simulink model "FirmwareController"  (R2022a)
settings: Solver=FixedStepDiscrete  StartTime=0.0  StopTime=10.0  RelTol=1e-3
model workspace (MAT data in the model file):
  HighLevel = Simulink.Bus
  HighLevel.Alignment = -1
  HighLevel.PreserveElementDimensions = 0
  HighLevel.Elements_internal(1) = Simulink.BusElement
  HighLevel.Elements_internal(1).DimensionsMode = 'Fixed'
  HighLevel.Elements_internal(1).SamplingMode = 'Sample based'
  HighLevel.Elements_internal(1).SampleTime = -1
  HighLevel.Elements_internal(1).Name = 'VelocityCommand'
  HighLevel.Elements_internal(1).DataType_internal = 'double'
  HighLevel.Elements_internal(1).Complexity = 'real'
  HighLevel.Elements_internal(1).Dimensions = 1
  HighLevel.Elements_internal(2) = Simulink.BusElement
  HighLevel.Elements_internal(2).DimensionsMode = 'Fixed'
  HighLevel.Elements_internal(2).SamplingMode = 'Sample based'
  HighLevel.Elements_internal(2).SampleTime = -1
  HighLevel.Elements_internal(2).Name = 'Odometry'
  HighLevel.Elements_internal(2).DataType_internal = 'double'
  HighLevel.Elements_internal(2).Complexity = 'real'
  HighLevel.Elements_internal(2).Dimensions = 1
  HighLevel.Elements_internal(3) = Simulink.BusElement
  HighLevel.Elements_internal(3).DimensionsMode = 'Fixed'
  HighLevel.Elements_internal(3).SamplingMode = 'Sample based'
  HighLevel.Elements_internal(3).SampleTime = -1
  HighLevel.Elements_internal(3).Name = 'ManipulatorTrajectory'
  HighLevel.Elements_internal(3).DataType_internal = 'double'
  HighLevel.Elements_internal(3).Complexity = 'real'
  HighLevel.Elements_internal(3).Dimensions = 1
  HighLevel.DataScope = 'Auto'
  ManipulatorSensorData = Simulink.Bus
  ManipulatorSensorData.Alignment = -1
  ManipulatorSensorData.PreserveElementDimensions = 0
  ManipulatorSensorData.Elements_internal(1) = Simulink.BusElement
  ManipulatorSensorData.Elements_internal(1).DimensionsMode = 'Fixed'
  ManipulatorSensorData.Elements_internal(1).SamplingMode = 'Sample based'
  ManipulatorSensorData.Elements_internal(1).SampleTime = -1
  ManipulatorSensorData.Elements_internal(1).Name = 'EncoderJoint1'
  ManipulatorSensorData.Elements_internal(1).DataType_internal = 'double'
  ManipulatorSensorData.Elements_internal(1).Complexity = 'real'
  ManipulatorSensorData.Elements_internal(1).Dimensions = 1
  ManipulatorSensorData.Elements_internal(2) = Simulink.BusElement
  ManipulatorSensorData.Elements_internal(2).DimensionsMode = 'Fixed'
  ManipulatorSensorData.Elements_internal(2).SamplingMode = 'Sample based'
  ManipulatorSensorData.Elements_internal(2).SampleTime = -1
  ManipulatorSensorData.Elements_internal(2).Name = 'EncoderJoint2'
  ManipulatorSensorData.Elements_internal(2).DataType_internal = 'double'
  ManipulatorSensorData.Elements_internal(2).Complexity = 'real'
  ManipulatorSensorData.Elements_internal(2).Dimensions = 1
  ManipulatorSensorData.Elements_internal(3) = Simulink.BusElement
  ManipulatorSensorData.Elements_internal(3).DimensionsMode = 'Fixed'
  ManipulatorSensorData.Elements_internal(3).SamplingMode = 'Sample based'
  ManipulatorSensorData.Elements_internal(3).SampleTime = -1
  ManipulatorSensorData.Elements_internal(3).Name = 'EncoderJoint3'
  ManipulatorSensorData.Elements_internal(3).DataType_internal = 'double'
  ManipulatorSensorData.Elements_internal(3).Complexity = 'real'
  ManipulatorSensorData.Elements_internal(3).Dimensions = 1
  ManipulatorSensorData.Elements_internal(4) = Simulink.BusElement
  ManipulatorSensorData.Elements_internal(4).DimensionsMode = 'Fixed'
  ManipulatorSensorData.Elements_internal(4).SamplingMode = 'Sample based'
  ManipulatorSensorData.Elements_internal(4).SampleTime = -1
  ManipulatorSensorData.Elements_internal(4).Name = 'EncoderJoint4'
  ManipulatorSensorData.Elements_internal(4).DataType_internal = 'double'
  ManipulatorSensorData.Elements_internal(4).Complexity = 'real'
  ManipulatorSensorData.Elements_internal(4).Dimensions = 1
  ManipulatorSensorData.Elements_internal(5) = Simulink.BusElement
  ManipulatorSensorData.Elements_internal(5).DimensionsMode = 'Fixed'
  ManipulatorSensorData.Elements_internal(5).SamplingMode = 'Sample based'
  ManipulatorSensorData.Elements_internal(5).SampleTime = -1
  ManipulatorSensorData.Elements_internal(5).Name = 'EncoderJoint5'
  ManipulatorSensorData.Elements_internal(5).DataType_internal = 'double'
  ManipulatorSensorData.Elements_internal(5).Complexity = 'real'
  ManipulatorSensorData.Elements_internal(5).Dimensions = 1
  ManipulatorSensorData.Elements_internal(6) = Simulink.BusElement
  ManipulatorSensorData.Elements_internal(6).DimensionsMode = 'Fixed'
  ManipulatorSensorData.Elements_internal(6).SamplingMode = 'Sample based'
  ManipulatorSensorData.Elements_internal(6).SampleTime = -1
  ManipulatorSensorData.Elements_internal(6).Name = 'EncoderJoint6'
  ManipulatorSensorData.Elements_internal(6).DataType_internal = 'double'
  ManipulatorSensorData.Elements_internal(6).Complexity = 'real'
  ManipulatorSensorData.Elements_internal(6).Dimensions = 1
  ManipulatorSensorData.Elements_internal(7) = Simulink.BusElement
  ManipulatorSensorData.Elements_internal(7).DimensionsMode = 'Fixed'
  ManipulatorSensorData.Elements_internal(7).SamplingMode = 'Sample based'
  ManipulatorSensorData.Elements_internal(7).SampleTime = -1
  ManipulatorSensorData.Elements_internal(7).Name = 'EncoderJoint7'
  ManipulatorSensorData.Elements_internal(7).DataType_internal = 'double'
  ManipulatorSensorData.Elements_internal(7).Complexity = 'real'
  ManipulatorSensorData.Elements_internal(7).Dimensions = 1
  ManipulatorSensorData.DataScope = 'Auto'
  MobileBaseSensorData = Simulink.Bus
  MobileBaseSensorData.Alignment = -1
  MobileBaseSensorData.PreserveElementDimensions = 0
  MobileBaseSensorData.Elements_internal(1) = Simulink.BusElement
  MobileBaseSensorData.Elements_internal(1).DimensionsMode = 'Fixed'
  MobileBaseSensorData.Elements_internal(1).SamplingMode = 'Sample based'
  MobileBaseSensorData.Elements_internal(1).SampleTime = -1
  MobileBaseSensorData.Elements_internal(1).Name = 'EncoderMotorL'
  MobileBaseSensorData.Elements_internal(1).DataType_internal = 'double'
  MobileBaseSensorData.Elements_internal(1).Complexity = 'real'
  MobileBaseSensorData.Elements_internal(1).Dimensions = 1
  MobileBaseSensorData.Elements_internal(2) = Simulink.BusElement
  MobileBaseSensorData.Elements_internal(2).DimensionsMode = 'Fixed'
  MobileBaseSensorData.Elements_internal(2).SamplingMode = 'Sample based'
  MobileBaseSensorData.Elements_internal(2).SampleTime = -1
  MobileBaseSensorData.Elements_internal(2).Name = 'EncoderMotorR'
  MobileBaseSensorData.Elements_internal(2).DataType_internal = 'double'
  MobileBaseSensorData.Elements_internal(2).Complexity = 'real'
  MobileBaseSensorData.Elements_internal(2).Dimensions = 1
  MobileBaseSensorData.Elements_internal(3) = Simulink.BusElement
  MobileBaseSensorData.Elements_internal(3).DimensionsMode = 'Fixed'
  MobileBaseSensorData.Elements_internal(3).SamplingMode = 'Sample based'
  MobileBaseSensorData.Elements_internal(3).SampleTime = -1
  MobileBaseSensorData.Elements_internal(3).Name = 'IMU'
  MobileBaseSensorData.Elements_internal(3).DataType_internal = 'double'
  MobileBaseSensorData.Elements_internal(3).Complexity = 'real'
  MobileBaseSensorData.Elements_internal(3).Dimensions = 1
  MobileBaseSensorData.DataScope = 'Auto'
settings Model: Creator=EarthPhisek  LastModifiedBy=EarthPhisek
settings OptimizationCC: EnhancedBackFolding=on  PassReuseOutputArgsAs=Individual arguments  ZeroExternalMemoryAtStartup=off  ZeroInternalMemoryAtStartup=off  MaxStackSize=64  OptimizeBlockOrder=speed  DifferentSizesBufferReuse=on  OptimizationCustomize=off  EfficientTunableParamExpr=on
settings DebuggingCC: ParameterTunabilityLossMsg=error
settings HardwareCC: UseEmbeddedCoderFeatures=off
settings SFSimCC: MATLABDynamicMemAlloc=off
settings RTWCC: SystemTargetFile=ert.tlc  HardwareBoard=Robot Operating System 2 (ROS 2)  TLCOptions="-aInlineSetEventsForThisBaseRateFcn=TLC_FALSE -aSuppressMultiTaskScheduler=TLC_FALSE  -aRateBasedStepFcn=0"  TemplateMakefile=ert_default_tmf  Toolchain=Colcon Tools  TargetLang=C++
settings CodeAppCC: ForceParamTrailComments=on  IgnoreCustomStorageClasses=off  OperatorAnnotations=on  SimulinkDataObjDesc=on  SFDataObjDesc=on  InsertBlockDesc=on
settings ERTTargetCC: CodeInterfacePackaging=C++ class  SupportNonInlinedSFcns=on  RootIOFormat=Structure reference

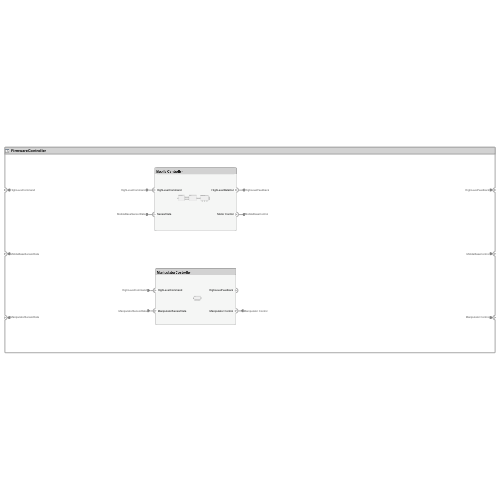
[thumbnail: Simulink's stored preview of the top-level diagram]
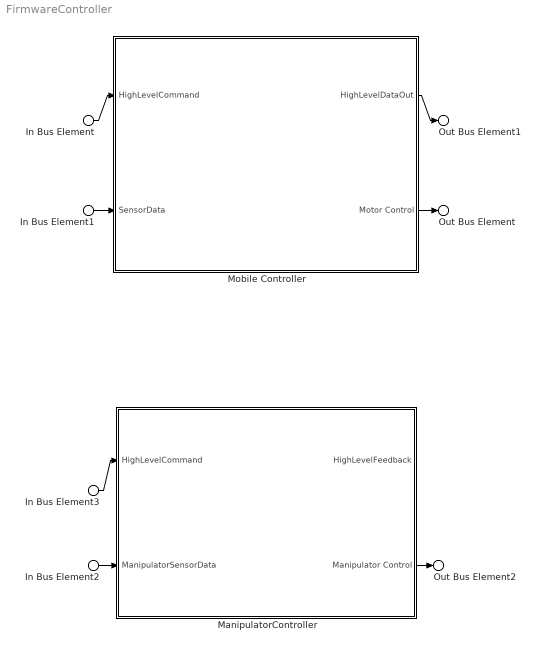
== system FirmwareController ==
  In Bus Element : Inport  PortName=HighLevelCommand
  In Bus Element3 : Inport  PortName=HighLevelCommand
  In Bus Element1 : Inport  Port=2  PortName=MobileBaseSensorData
  In Bus Element2 : Inport  Port=3  PortName=ManipulatorSensorData
  ManipulatorController : Subsystem
      settings: PortSchema="{\"entries\":[{\"content\":{\"headerSize\":26,\"margin\":15,\"minimumSpacing\":25,\"sides\":[{\"content\":{\"connectorIds\":[\"In1\",\"In2\"]},\"type\":\"ConnectorPlacement.EquallySpacedRectSide\",\"uuid\":\"c98ff4be-64d0-449e-9b1d-a8301930c005\"},{\"content\":{\"connectorIds\":[\"Out1\",\"Out2\"],\"side\":\"RIGHT\"},\"type\":\"ConnectorPlacement.EquallySpacedRectSide\",\"uuid\":\"687eed08-6ff3-4e87-827e-4ed9dc740528\"},{\"content\":{\"connectorIds\":[],\"side\":\"TOP\"},\"type\":\"ConnectorPlacement.EquallySpacedRectSide\",\"uuid\":\"c1e53efb-7b04-4802-8059-06db2c482b4f\"}]},\"type\":\"ConnectorPlacement.EquallySpacedConnector\",\"uuid\":\"21e22d49-20f6-4ec3-b79a-f2c75a9aa23d\"}],\"packageUris\":[\"http://schema.mathworks.com/mf0/Connector/R2020b\"],\"version\":\"1.0\"}"
  Mobile Controller : Subsystem
      settings: PortSchema="{\"entries\":[{\"content\":{\"headerSize\":26,\"margin\":15,\"minimumSpacing\":25,\"sides\":[{\"content\":{\"connectorIds\":[\"In1\",\"In2\"]},\"type\":\"ConnectorPlacement.EquallySpacedRectSide\",\"uuid\":\"dd41dd12-49ec-4c74-984d-ae398e001f17\"},{\"content\":{\"connectorIds\":[\"Out1\",\"Out2\"],\"side\":\"RIGHT\"},\"type\":\"ConnectorPlacement.EquallySpacedRectSide\",\"uuid\":\"7b6711d5-260d-4adb-8390-dd0a2fe64eed\"},{\"content\":{\"connectorIds\":[],\"side\":\"TOP\"},\"type\":\"ConnectorPlacement.EquallySpacedRectSide\",\"uuid\":\"51c2854e-5efe-4dec-8c07-70731026f3e8\"}]},\"type\":\"ConnectorPlacement.EquallySpacedConnector\",\"uuid\":\"aa3377b9-5458-4828-a095-24c10dd42ea0\"}],\"packageUris\":[\"http://schema.mathworks.com/mf0/Connector/R2020b\"],\"version\":\"1.0\"}"
  Out Bus Element1 : Outport  PortName=HighLevelFeedback
  Out Bus Element : Outport  Port=2  PortName=MobileBaseControl
  Out Bus Element2 : Outport  Port=3  PortName=Manipulator Control
  wires:
  In Bus Element1/1 -> Mobile Controller/2(SensorData)
  In Bus Element/1 -> Mobile Controller/1(HighLevelCommand)
  In Bus Element2/1 -> ManipulatorController/2(ManipulatorSensorData)
  In Bus Element3/1 -> ManipulatorController/1(HighLevelCommand)
  Mobile Controller/2(Motor Control) -> Out Bus Element/1
  Mobile Controller/1(HighLevelDataOut) -> Out Bus Element1/1
  ManipulatorController/2(Manipulator Control) -> Out Bus Element2/1

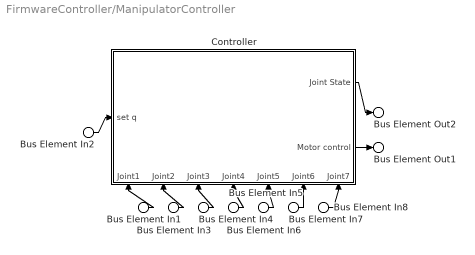
== system FirmwareController/ManipulatorController ==
  Bus Element In2 : Inport  PortName=HighLevelCommand  Element=ManipulatorTrajectory
  Bus Element In1 : Inport  Port=2  PortName=ManipulatorSensorData  Element=EncoderJoint1
  Bus Element In3 : Inport  Port=2  PortName=ManipulatorSensorData  Element=EncoderJoint2
  Bus Element In4 : Inport  Port=2  PortName=ManipulatorSensorData  Element=EncoderJoint3
  Bus Element In5 : Inport  Port=2  PortName=ManipulatorSensorData  Element=EncoderJoint4
  Bus Element In6 : Inport  Port=2  PortName=ManipulatorSensorData  Element=EncoderJoint5
  Bus Element In7 : Inport  Port=2  PortName=ManipulatorSensorData  Element=EncoderJoint6
  Bus Element In8 : Inport  Port=2  PortName=ManipulatorSensorData  Element=EncoderJoint7
  Controller : Subsystem
      settings: PortSchema="{\"entries\":[{\"content\":{\"headerSize\":26,\"margin\":15,\"minimumSpacing\":25,\"sides\":[{\"content\":{\"connectorIds\":[\"In8\"]},\"type\":\"ConnectorPlacement.EquallySpacedRectSide\",\"uuid\":\"c98ff4be-64d0-449e-9b1d-a8301930c005\"},{\"content\":{\"connectorIds\":[\"Out1\",\"Out2\"],\"side\":\"RIGHT\"},\"type\":\"ConnectorPlacement.EquallySpacedRectSide\",\"uuid\":\"687eed08-6ff3-4e87-827e-4ed9dc740528\"},{\"content\":{\"connectorIds\":[],\"side\":\"TOP\"},\"type\":\"ConnectorPlacement.EquallySpacedRectSide\",\"uuid\":\"c1e53efb-7b04-4802-8059-06db2c482b4f\"},{\"content\":{\"connectorIds\":[\"In1\",\"In2\",\"In3\",\"In4\",\"In5\",\"In6\",\"In7\"],\"side\":\"BOTTOM\"},\"type\":\"ConnectorPlacement.EquallySpacedRectSide\",\"uuid\":\"95d433fb-5879-44e1-b6c3-cfb52e1509f1\"}]},\"type\":\"ConnectorPlacement.EquallySpacedConnector\",\"uuid\":\"21e22d49-20f6-4ec3-b79a-f2c75a9aa23d\"}],\"packageUris\":[\"http://schema.mathworks.com/mf0/Connector/R2020b\"],\"version\":\"1.0\"}"
  Bus Element Out2 : Outport  PortName=HighLevelFeedback
  Bus Element Out1 : Outport  Port=2  PortName=Manipulator Control
  wires:
  Bus Element In1/1 -> Controller/1(Joint1)
  Bus Element In3/1 -> Controller/2(Joint2)
  Bus Element In4/1 -> Controller/3(Joint3)
  Bus Element In5/1 -> Controller/4(Joint4)
  Bus Element In6/1 -> Controller/5(Joint5)
  Bus Element In7/1 -> Controller/6(Joint6)
  Bus Element In8/1 -> Controller/7(Joint7)
  Controller/2(Motor control) -> Bus Element Out1/1
  Controller/1(Joint State) -> Bus Element Out2/1
  Bus Element In2/1 -> Controller/8("set q ")

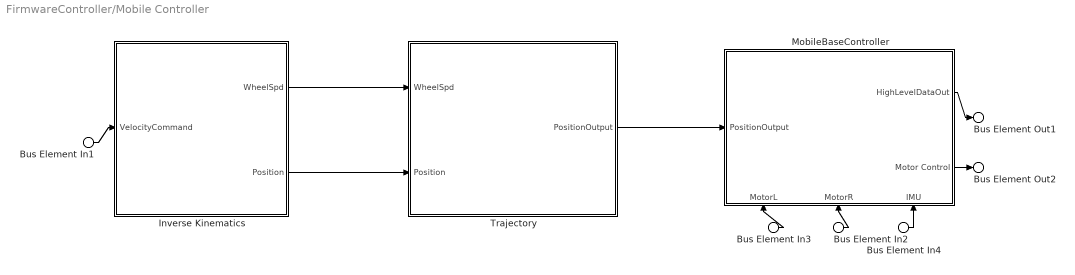
== system FirmwareController/Mobile Controller ==
  Bus Element In1 : Inport  PortName=HighLevelCommand  Element=VelocityCommand
  Bus Element In3 : Inport  Port=2  PortName=SensorData  Element=EncoderMotorL
  Bus Element In2 : Inport  Port=2  PortName=SensorData  Element=EncoderMotorR
  Bus Element In4 : Inport  Port=2  PortName=SensorData  Element=IMU
  Inverse Kinematics : Subsystem
      settings: PortSchema="{\"entries\":[{\"content\":{\"headerSize\":26,\"margin\":15,\"minimumSpacing\":25,\"sides\":[{\"content\":{\"connectorIds\":[\"In1\"]},\"type\":\"ConnectorPlacement.EquallySpacedRectSide\",\"uuid\":\"c98ff4be-64d0-449e-9b1d-a8301930c005\"},{\"content\":{\"connectorIds\":[\"Out1\",\"Out2\"],\"side\":\"RIGHT\"},\"type\":\"ConnectorPlacement.EquallySpacedRectSide\",\"uuid\":\"687eed08-6ff3-4e87-827e-4ed9dc740528\"},{\"content\":{\"connectorIds\":[],\"side\":\"TOP\"},\"type\":\"ConnectorPlacement.EquallySpacedRectSide\",\"uuid\":\"c1e53efb-7b04-4802-8059-06db2c482b4f\"}]},\"type\":\"ConnectorPlacement.EquallySpacedConnector\",\"uuid\":\"21e22d49-20f6-4ec3-b79a-f2c75a9aa23d\"}],\"packageUris\":[\"http://schema.mathworks.com/mf0/Connector/R2020b\"],\"version\":\"1.0\"}"
  MobileBaseController : Subsystem
      settings: PortSchema="{\"entries\":[{\"content\":{\"headerSize\":26,\"margin\":15,\"minimumSpacing\":25,\"sides\":[{\"content\":{\"connectorIds\":[\"In4\"]},\"type\":\"ConnectorPlacement.EquallySpacedRectSide\",\"uuid\":\"c98ff4be-64d0-449e-9b1d-a8301930c005\"},{\"content\":{\"connectorIds\":[\"Out1\",\"Out2\"],\"side\":\"RIGHT\"},\"type\":\"ConnectorPlacement.EquallySpacedRectSide\",\"uuid\":\"687eed08-6ff3-4e87-827e-4ed9dc740528\"},{\"content\":{\"connectorIds\":[],\"side\":\"TOP\"},\"type\":\"ConnectorPlacement.EquallySpacedRectSide\",\"uuid\":\"c1e53efb-7b04-4802-8059-06db2c482b4f\"},{\"content\":{\"connectorIds\":[\"In1\",\"In2\",\"In3\"],\"side\":\"BOTTOM\"},\"type\":\"ConnectorPlacement.EquallySpacedRectSide\",\"uuid\":\"72bc73f6-9a9a-4420-89c6-6eb47a518707\"}]},\"type\":\"ConnectorPlacement.EquallySpacedConnector\",\"uuid\":\"21e22d49-20f6-4ec3-b79a-f2c75a9aa23d\"}],\"packageUris\":[\"http://schema.mathworks.com/mf0/Connector/R2020b\"],\"version\":\"1.0\"}"
  Trajectory : Subsystem
      settings: PortSchema="{\"entries\":[{\"content\":{\"headerSize\":26,\"margin\":15,\"minimumSpacing\":25,\"sides\":[{\"content\":{\"connectorIds\":[\"In1\",\"In2\"]},\"type\":\"ConnectorPlacement.EquallySpacedRectSide\",\"uuid\":\"c98ff4be-64d0-449e-9b1d-a8301930c005\"},{\"content\":{\"connectorIds\":[\"Out1\"],\"side\":\"RIGHT\"},\"type\":\"ConnectorPlacement.EquallySpacedRectSide\",\"uuid\":\"687eed08-6ff3-4e87-827e-4ed9dc740528\"},{\"content\":{\"connectorIds\":[],\"side\":\"TOP\"},\"type\":\"ConnectorPlacement.EquallySpacedRectSide\",\"uuid\":\"c1e53efb-7b04-4802-8059-06db2c482b4f\"}]},\"type\":\"ConnectorPlacement.EquallySpacedConnector\",\"uuid\":\"21e22d49-20f6-4ec3-b79a-f2c75a9aa23d\"}],\"packageUris\":[\"http://schema.mathworks.com/mf0/Connector/R2020b\"],\"version\":\"1.0\"}"
  Bus Element Out1 : Outport  PortName=HighLevelDataOut  Element=Odometry
  Bus Element Out2 : Outport  Port=2  PortName=Motor Control
  wires:
  Bus Element In1/1 -> Inverse Kinematics/1(VelocityCommand)
  Inverse Kinematics/1(WheelSpd) -> Trajectory/1(WheelSpd)
  Inverse Kinematics/2(Position) -> Trajectory/2(Position)
  Trajectory/1(PositionOutput) -> MobileBaseController/4(PositionOutput)
  Bus Element In3/1 -> MobileBaseController/1(MotorL)
  Bus Element In2/1 -> MobileBaseController/2(MotorR)
  Bus Element In4/1 -> MobileBaseController/3(IMU)
  MobileBaseController/2(Motor Control) -> Bus Element Out2/1
  MobileBaseController/1(HighLevelDataOut) -> Bus Element Out1/1

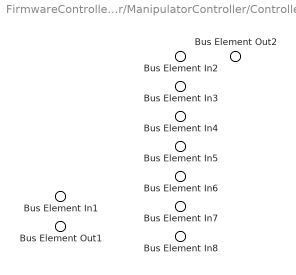
== system FirmwareController/ManipulatorController/Controller ==
  Bus Element In2 : Inport  PortName=Joint1
  Bus Element In3 : Inport  Port=2  PortName=Joint2
  Bus Element In4 : Inport  Port=3  PortName=Joint3
  Bus Element In5 : Inport  Port=4  PortName=Joint4
  Bus Element In6 : Inport  Port=5  PortName=Joint5
  Bus Element In7 : Inport  Port=6  PortName=Joint6
  Bus Element In8 : Inport  Port=7  PortName=Joint7
  Bus Element In1 : Inport  Port=8  PortName=set q
  Bus Element Out2 : Outport  PortName=Joint State
  Bus Element Out1 : Outport  Port=2  PortName=Motor control

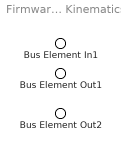
== system FirmwareController/Mobile Controller/Inverse Kinematics ==
  Bus Element In1 : Inport  PortName=VelocityCommand
  Bus Element Out1 : Outport  PortName=WheelSpd
  Bus Element Out2 : Outport  Port=2  PortName=Position

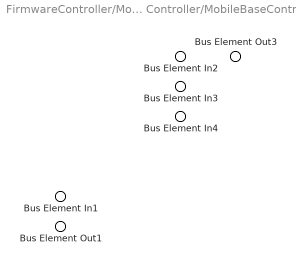
== system FirmwareController/Mobile Controller/MobileBaseController ==
  Bus Element In2 : Inport  PortName=MotorL
  Bus Element In3 : Inport  Port=2  PortName=MotorR
  Bus Element In4 : Inport  Port=3  PortName=IMU
  Bus Element In1 : Inport  Port=4  PortName=PositionOutput
  Bus Element Out3 : Outport  PortName=HighLevelDataOut
  Bus Element Out1 : Outport  Port=2  PortName=Motor Control

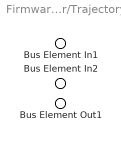
== system FirmwareController/Mobile Controller/Trajectory ==
  Bus Element In1 : Inport  PortName=WheelSpd
  Bus Element In2 : Inport  Port=2  PortName=Position
  Bus Element Out1 : Outport  PortName=PositionOutput
